simulink model "Child"  (R2023a)
settings: Solver=FixedStepAuto  StartTime=0.0  StopTime=inf  RelTol=1e-3
undefined symbols (not defined in the file): Alert1, Boolean_Value, DiscIntNeverNeededParam, JAN, Speed, Value_, X
libraries: androidcommunicationlib x4, androiduilib x4, androidsensorlib x3, androidaudiovideolib x3
settings Model: Creator=nishi  LastModifiedBy=abhimanyuyadav
settings OptimizationCC: EnhancedBackFolding=on  PassReuseOutputArgsAs=Individual arguments  ZeroExternalMemoryAtStartup=off  ZeroInternalMemoryAtStartup=off  MaxStackSize=64  SimCompilerOptimization=on  OptimizeBlockOrder=speed  DifferentSizesBufferReuse=on  OptimizationCustomize=off  EfficientTunableParamExpr=on
settings DebuggingCC: ParameterPrecisionLossMsg=none  ParameterTunabilityLossMsg=error
settings HardwareCC: ProdBitPerPointer=32  ProdBitPerSizeT=32  ProdBitPerPtrDiffT=32  ProdLargestAtomicInteger=Long  ProdLargestAtomicFloat=Double  ProdWordSize=32  ProdHWDeviceType=ARM Compatible->ARM Cortex
settings SFSimCC: MATLABDynamicMemAlloc=off
settings RTWCC: Description=Embedded Coder  SystemTargetFile=ert.tlc  HardwareBoard=Android Device  TLCOptions="-aInlineSetEventsForThisBaseRateFcn=TLC_FALSE -aSuppressMultiTaskScheduler=TLC_FALSE  -aRateBasedStepFcn=0"  TemplateMakefile=ert_default_tmf  RTWVerbose=off  Toolchain=Android SDK/NDK Tools
settings CodeAppCC: ForceParamTrailComments=on  IgnoreCustomStorageClasses=off  OperatorAnnotations=on  SimulinkDataObjDesc=on  SFDataObjDesc=on  InsertBlockDesc=on
settings ERTTargetCC: SupportNonInlinedSFcns=on

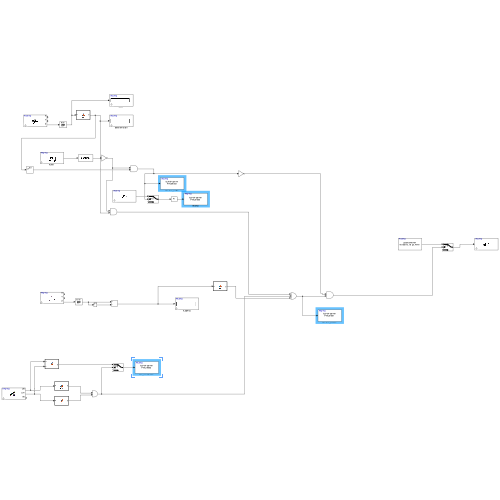
[thumbnail: Simulink's stored preview of the top-level diagram]
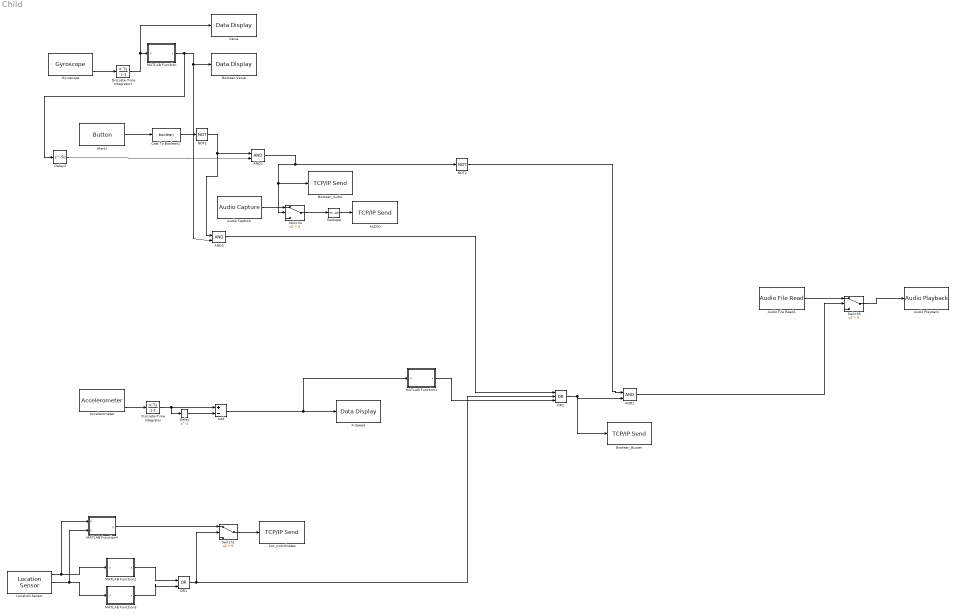
== system Child ==
  AND1 : Logic  IconShape=distinctive  AllPortsSameDT=off  OutDataTypeStr=boolean
  AND2 : Logic  IconShape=distinctive  AllPortsSameDT=off  OutDataTypeStr=boolean
  AND3 : Logic  IconShape=distinctive  AllPortsSameDT=off  OutDataTypeStr=boolean
  AUDIO : androidcommunicationlib/TCP//IP Send  TCPSendId=JAN/TCP//IP_Send  Mode_=Server  LocalServerPort_=39000  RemoteAddr_=10.7.10.145  RemoteServerPort_=39000  ClientPortBindingSelection_=off  ClientPortToBind_=35000  BlockingMode_=off  BlockTimeout_=0.1
  Accelerometer : androidsensorlib/Accelerometer  OutputVector=off  SampleTime=0.1  BlockPlatform=Android
  Add : Sum  Inputs=+-
  Alert1 : androiduilib/Button  ButtonState=Not pressed  ButtonId=JAN/Alert1  State=off  SampleTime=0.1  BlockPlatform=Android
  Audio Capture : androidaudiovideolib/Audio Capture  SampleFreq=44100  FrameSize=4410  SampleTime=0.1  SimulateUsing=Code generation  DeviceStr=0  QueueDuration=0  BlockPlatform=Android  AudioSamplingFreq=44100
  Audio File Read1 : androidaudiovideolib/Audio File Read  FileName=C:\Users\DELL\Downloads\emergency-alarm-with-reverb-29431.mp3  FrameSize=2400
  Audio Playback : androidaudiovideolib/Audio Playback  SampleFreq=24000  AudioSamplingFreq=24000  SampleTime=0.1  DeviceStr=0  QueueDuration=0  BlockPlatform=Android
  Boolean Value : androiduilib/Data Display  DataDisplayId=JAN/Boolean_Value  Format=Float  Precision=6  SimulateUsing=Code generation  blockPlatform=Android
  Boolean_Audio : androidcommunicationlib/TCP//IP Send  TCPSendId=JAN/TCP//IP_Send  Mode_=Server  LocalServerPort_=39003  RemoteAddr_=10.7.10.145  RemoteServerPort_=39000  ClientPortBindingSelection_=off  ClientPortToBind_=35000  BlockingMode_=off  BlockTimeout_=0.1
  Boolean_Buzzer : androidcommunicationlib/TCP//IP Send  Mode_=Server  LocalServerPort_=39001  RemoteAddr_=127.0.0.1  RemoteServerPort_=25000  ClientPortBindingSelection_=off  ClientPortToBind_=35000  BlockingMode_=off  BlockTimeout_=0.1
  Cast To Boolean1 : DataTypeConversion  OutDataTypeStr=boolean  SaturateOnIntegerOverflow=off  RndMeth=Floor
  Delay : Delay  DelayLength=1  InitialCondition=0
  Delay2 : Delay  DelayLength=50  InitialCondition=0
  Discrete-Time Integrator : DiscreteIntegrator  SampleTime=-1  ICPrevOutput=DiscIntNeverNeededParam  ICPrevScaledInput=DiscIntNeverNeededParam
  Discrete-Time Integrator1 : DiscreteIntegrator  SampleTime=-1  ICPrevOutput=DiscIntNeverNeededParam  ICPrevScaledInput=DiscIntNeverNeededParam
  Gyroscope : androidsensorlib/Gyroscope  OutputVector=off  SampleTime=0.1  BlockPlatform=Android
  Loc_coordinates : androidcommunicationlib/TCP//IP Send  Mode_=Server  LocalServerPort_=39002  RemoteAddr_=127.0.0.1  RemoteServerPort_=25000  ClientPortBindingSelection_=off  ClientPortToBind_=35000  BlockingMode_=off  BlockTimeout_=0.1
  Location Sensor : androidsensorlib/Location Sensor  OutputVector=off  SampleTime=0.1  BlockPlatform=Android
  MATLAB Function : MATLAB Function  TreatAsAtomicUnit=on
  MATLAB Function1 : MATLAB Function  TreatAsAtomicUnit=on
  MATLAB Function2 : MATLAB Function  TreatAsAtomicUnit=on
  MATLAB Function3 : MATLAB Function  TreatAsAtomicUnit=on
  MATLAB Function4 : MATLAB Function  TreatAsAtomicUnit=on
  NOT1 : Logic  Operator=NOT  IconShape=distinctive  AllPortsSameDT=off  OutDataTypeStr=boolean
  NOT2 : Logic  Operator=NOT  IconShape=distinctive  AllPortsSameDT=off  OutDataTypeStr=boolean
  OR1 : Logic  Operator=OR  IconShape=distinctive  AllPortsSameDT=off  OutDataTypeStr=boolean
  OR2 : Logic  Operator=OR  Inputs=3  IconShape=distinctive  AllPortsSameDT=off  OutDataTypeStr=boolean
  Reshape : Reshape  OutputDimensionality=Customize  OutputDimensions=[8820,1]
  Switch1 : Switch  Criteria=u2 > Threshold  SaturateOnIntegerOverflow=off  InputSameDT=off
  Switch4 : Switch  Criteria=u2 > Threshold  SaturateOnIntegerOverflow=off  InputSameDT=off
  Switch5 : Switch  Criteria=u2 > Threshold  SaturateOnIntegerOverflow=off  InputSameDT=off
  "Value " : androiduilib/Data Display  DataDisplayId=JAN/Value_  Format=Float  Precision=6  SimulateUsing=Code generation  blockPlatform=Android
  X-Speed : androiduilib/Data Display  DataDisplayId=JAN/X-Speed  Format=Float  Precision=6  SimulateUsing=Code generation  blockPlatform=Android
  wires:
  Audio File Read1/1 -> Switch5/1
  MATLAB Function3/1(y) -> OR1/2
  Location Sensor/1 -> MATLAB Function4/1(u), MATLAB Function2/1(u)
  MATLAB Function2/1(y) -> OR1/1
  Switch5/1 -> Audio Playback/1
  Discrete-Time Integrator1/1 -> "Value "/1, MATLAB Function/1(u)
  Location Sensor/2 -> MATLAB Function4/2(v), MATLAB Function3/1(u)
  Add/1 -> MATLAB Function1/1(u), X-Speed/1
  Alert1/1 -> Cast To Boolean1/1
  NOT1/1 -> AND3/1, AND2/1
  AND2/1 -> NOT2/1, Boolean_Audio/1, Switch4/2
  Cast To Boolean1/1 -> NOT1/1
  Delay2/1 -> AND2/2
  NOT2/1 -> AND1/1
  MATLAB Function/1(y) -> AND3/2, Boolean Value/1, Delay2/1
  OR2/1 -> Boolean_Buzzer/1, AND1/2
  AND3/1 -> OR2/1
  OR1/1 -> Switch1/2, OR2/2
  AND1/1 -> Switch5/2
  Reshape/1 -> AUDIO/1
  Audio Capture/1 -> Switch4/1
  Switch4/1 -> Reshape/1
  Delay/1 -> Add/2
  Accelerometer/3 -> Discrete-Time Integrator/1
  Discrete-Time Integrator/1 -> Delay/1, Add/1
  MATLAB Function1/1(y) -> OR2/3
  Gyroscope/3 -> Discrete-Time Integrator1/1
  Switch1/1 -> Loc_coordinates/1
  MATLAB Function4/1(y) -> Switch1/1

== matlab function Child/MATLAB Function ==
  data: u input; y output
function y = fcn(u)

if u > 1.6
    y = true;
else
    y = false;
end
end

== matlab function Child/MATLAB Function4 ==
  data: u input; y output; v input
function y = fcn(u,v)

y=[u,v];
end

== matlab function Child/MATLAB Function2 ==
  data: u input; y output
function y = fcn(u)

if (u > 23.210 && u<23.211)
    y = false;
else
    y = true;
end
end

== matlab function Child/MATLAB Function3 ==
  data: u input; y output
function y = fcn(u)

if (u > 72.685 && u<72.686)
    y = false;
else
    y = true;
end
end

== matlab function Child/MATLAB Function1 ==
  data: u input; y output
function y = fcn(u)

if u > 0.2
    y = true;
else
    y = false;
end
end
